simulink model "arquitetura"  (R2021a)
settings: Solver=VariableStepAuto  StartTime=0.0  StopTime=Ttotal  RelTol=1e-20
values from neighbouring files (symbols this model uses):
  r = R'*(current-reference)    [implemented_controller.m]
undefined symbols (not defined in the file or in its folder): def_seed, DiscIntNeverNeededParam, drone1_psi0, drone1_v0, drone1_x0, drone1_y0, drone2_psi0, drone2_v0, drone2_x0, drone2_y0, drone3_psi0, drone3_v0, drone3_x0, drone3_y0, gama_dot_constant, max_psi, max_vel, min_psi, min_vel, N, target_velocity, Ts, vel_target, vel_target_x, x0, y0
libraries: commrandsrc3 x2
settings Model: Creator=migue  LastModifiedBy=migue

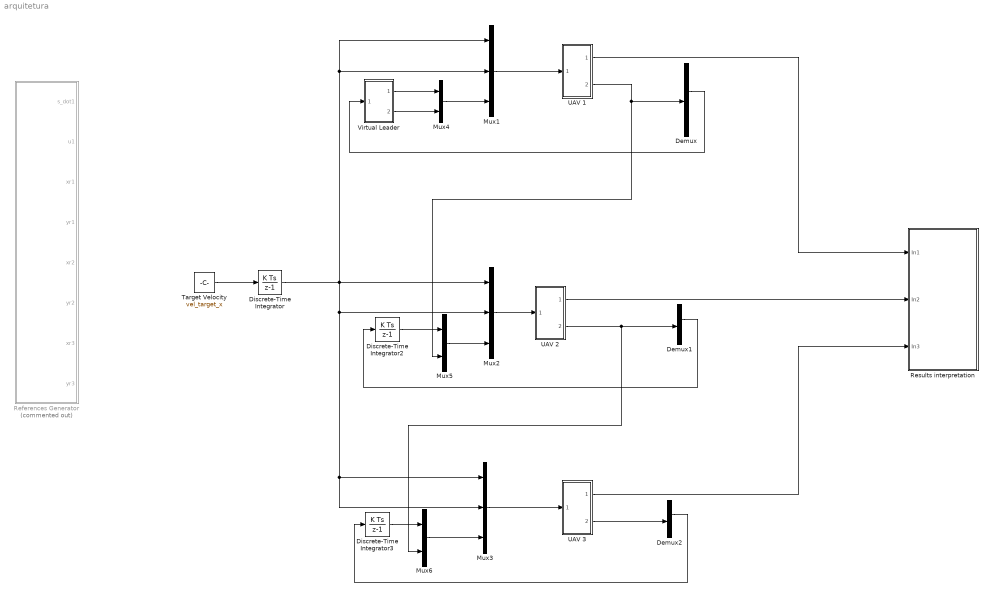
== system arquitetura ==
  Demux : Demux
  Demux1 : Demux
  Demux2 : Demux
  Discrete-Time Integrator : DiscreteIntegrator  SampleTime=Ts  ICPrevOutput=DiscIntNeverNeededParam  ICPrevScaledInput=DiscIntNeverNeededParam
  Discrete-Time Integrator2 : DiscreteIntegrator  SampleTime=Ts  ICPrevOutput=DiscIntNeverNeededParam  ICPrevScaledInput=DiscIntNeverNeededParam
  Discrete-Time Integrator3 : DiscreteIntegrator  SampleTime=Ts  ICPrevOutput=DiscIntNeverNeededParam  ICPrevScaledInput=DiscIntNeverNeededParam
  Mux1 : Mux  Inputs=3
  Mux2 : Mux  Inputs=3
  Mux3 : Mux  Inputs=3
  Mux4 : Mux  Inputs=2
  Mux5 : Mux  Inputs=2
  Mux6 : Mux  Inputs=2
  References Generator : Subsystem  Commented=on
  Results interpretation : Subsystem
  Target Velocity : Constant  Value=vel_target_x  SampleTime=Ts
  UAV 1 : Subsystem
  UAV 2 : Subsystem
  UAV 3 : Subsystem
  Virtual Leader : Subsystem
  wires:
  Mux1/1 -> UAV 1/1((x;y))
  Mux2/1 -> UAV 2/1((x;y))
  Mux3/1 -> UAV 3/1((x;y))
  Discrete-Time Integrator/1 -> Mux1/1, Mux1/2, Mux2/1, Mux3/2, Mux3/1, Mux2/2
  Target Velocity/1 -> Discrete-Time Integrator/1
  Mux4/1 -> Mux1/3
  UAV 1/2(Output) -> Demux/1, Mux5/2
  Discrete-Time Integrator2/1 -> Mux5/1
  Mux5/1 -> Mux2/3
  UAV 2/2(Output) -> Mux6/2, Demux1/1
  Mux6/1 -> Mux3/3
  Discrete-Time Integrator3/1 -> Mux6/1
  UAV 3/2(Output) -> Demux2/1
  UAV 1/1(Out1) -> Results interpretation/1(In1)
  UAV 2/1(Out1) -> Results interpretation/2(In2)
  UAV 3/1(Out1) -> Results interpretation/3(In3)
  Virtual Leader/1(Out1) -> Mux4/1
  Virtual Leader/2(Out2) -> Mux4/2
  Demux/2 -> Virtual Leader/1(Input)
  Demux1/2 -> Discrete-Time Integrator2/1
  Demux2/2 -> Discrete-Time Integrator3/1

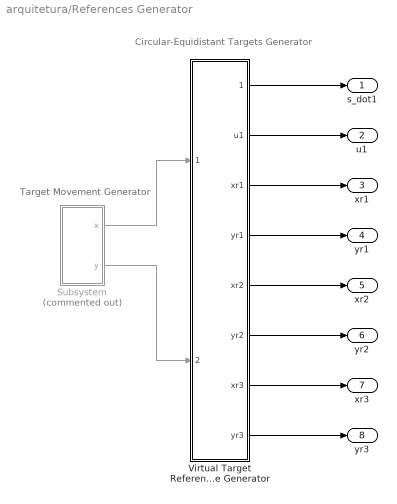
== system arquitetura/References Generator ==
  note: Target Movement Generator
  note: Circular-Equidistant Targets Generator
  Subsystem : Subsystem  Commented=on
  Virtual Target Reference Generator : Subsystem
  s_dot1 : Outport
  u1 : Outport  Port=2
  xr1 : Outport  Port=3
  yr1 : Outport  Port=4
  xr2 : Outport  Port=5
  yr2 : Outport  Port=6
  xr3 : Outport  Port=7
  yr3 : Outport  Port=8
  wires:
  Subsystem/2(y) -> Virtual Target Reference Generator/2(Input1)
  Subsystem/1(x) -> Virtual Target Reference Generator/1(Input)
  Virtual Target Reference Generator/4(yr1) -> yr1/1
  Virtual Target Reference Generator/6(yr2) -> yr2/1
  Virtual Target Reference Generator/3(xr1) -> xr1/1
  Virtual Target Reference Generator/5(xr2) -> xr2/1
  Virtual Target Reference Generator/8(yr3) -> yr3/1
  Virtual Target Reference Generator/7(xr3) -> xr3/1
  Virtual Target Reference Generator/2(u1) -> u1/1
  Virtual Target Reference Generator/1(s_dot1) -> s_dot1/1

== system arquitetura/Results interpretation ==
  In1 : Inport
  In2 : Inport  Port=2
  In3 : Inport  Port=3
  Draws Results : MATLABFcn  MATLABFcn=draw_results  OutputDimensions=0
  Mux : Mux  Inputs=3
  To Workspace : ToWorkspace  VariableName=simulation_data  SampleTime=-1
  wires:
  Mux/1 -> To Workspace/1, Draws Results/1
  In3/1 -> Mux/3
  In2/1 -> Mux/2
  In1/1 -> Mux/1

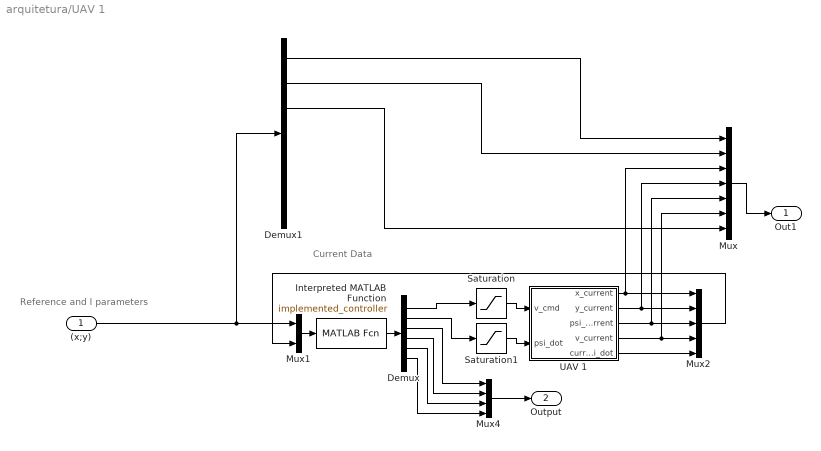
== system arquitetura/UAV 1 ==
  note: Current Data
  note: Reference and l parameters
  (x;y) : Inport
  Demux : Demux  Outputs=6
  Demux1 : Demux  Outputs=7
  Interpreted MATLAB Function : MATLABFcn  MATLABFcn=implemented_controller  OutputDimensions=6
  Mux : Mux  Inputs=7
  Mux1 : Mux  Inputs=2
  Mux2 : Mux  Inputs=5
  Mux4 : Mux
  Saturation : Saturate  UpperLimit=max_vel  LowerLimit=min_vel
  Saturation1 : Saturate  UpperLimit=max_psi  LowerLimit=min_psi
  UAV 1 : Subsystem
  Out1 : Outport
  Output : Outport  Port=2
  wires:
  Mux1/1 -> Interpreted MATLAB Function/1
  Interpreted MATLAB Function/1 -> Demux/1
  Demux/1 -> Saturation/1
  Saturation1/1 -> UAV 1/2(psi_dot)
  UAV 1/4(v_current) -> Mux/6, Mux2/4
  Mux2/1 -> Mux1/2
  Saturation/1 -> UAV 1/1(v_cmd)
  Demux/2 -> Saturation1/1
  (x;y)/1 -> Demux1/1, Mux1/1
  Demux1/1 -> Mux/1
  Demux1/2 -> Mux/2
  Mux/1 -> Out1/1
  UAV 1/3(psi_current) -> Mux/5, Mux2/3
  UAV 1/1(x_current) -> Mux/3, Mux2/1
  UAV 1/2(y_current) -> Mux/4, Mux2/2
  Demux/3 -> Mux4/1
  Demux/4 -> Mux4/2
  Mux4/1 -> Output/1
  Demux/5 -> Mux4/3
  Demux/6 -> Mux4/4
  UAV 1/5(current_psi_dot) -> Mux2/5
  Demux1/3 -> Mux/7

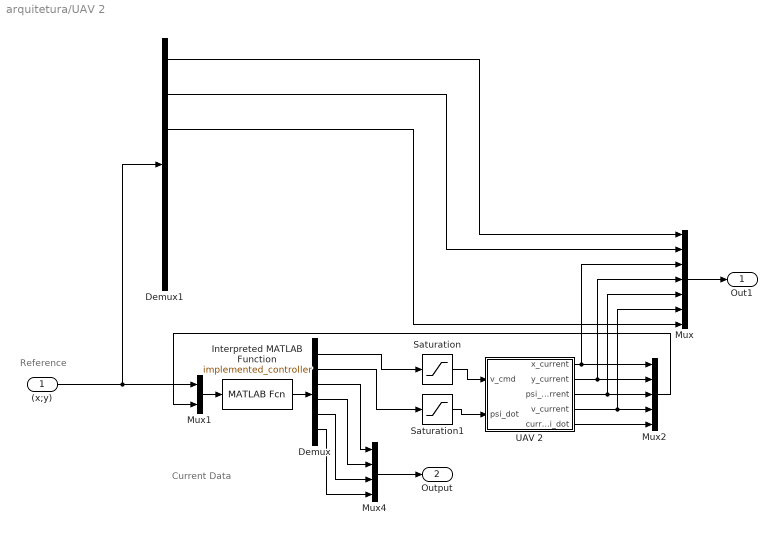
== system arquitetura/UAV 2 ==
  note: Current Data
  note: Reference
  (x;y) : Inport
  Demux : Demux  Outputs=6
  Demux1 : Demux  Outputs=7
  Interpreted MATLAB Function : MATLABFcn  MATLABFcn=implemented_controller  OutputDimensions=6
  Mux : Mux  Inputs=7
  Mux1 : Mux  Inputs=2
  Mux2 : Mux  Inputs=5
  Mux4 : Mux
  Saturation : Saturate  UpperLimit=max_vel  LowerLimit=min_vel
  Saturation1 : Saturate  UpperLimit=max_psi  LowerLimit=min_psi
  UAV 2 : Subsystem
  Out1 : Outport
  Output : Outport  Port=2
  wires:
  UAV 2/3(psi_current) -> Mux/5, Mux2/3
  Mux1/1 -> Interpreted MATLAB Function/1
  UAV 2/1(x_current) -> Mux2/1, Mux/3
  Interpreted MATLAB Function/1 -> Demux/1
  Demux/1 -> Saturation/1
  Saturation1/1 -> UAV 2/2(psi_dot)
  UAV 2/2(y_current) -> Mux/4, Mux2/2
  UAV 2/4(v_current) -> Mux/6, Mux2/4
  Mux2/1 -> Mux1/2
  Demux/2 -> Saturation1/1
  (x;y)/1 -> Demux1/1, Mux1/1
  Demux1/1 -> Mux/1
  Demux1/2 -> Mux/2
  Mux/1 -> Out1/1
  Mux4/1 -> Output/1
  Demux/3 -> Mux4/1
  Demux/4 -> Mux4/2
  Demux/5 -> Mux4/3
  Demux/6 -> Mux4/4
  Saturation/1 -> UAV 2/1(v_cmd)
  UAV 2/5(current_psi_dot) -> Mux2/5
  Demux1/3 -> Mux/7

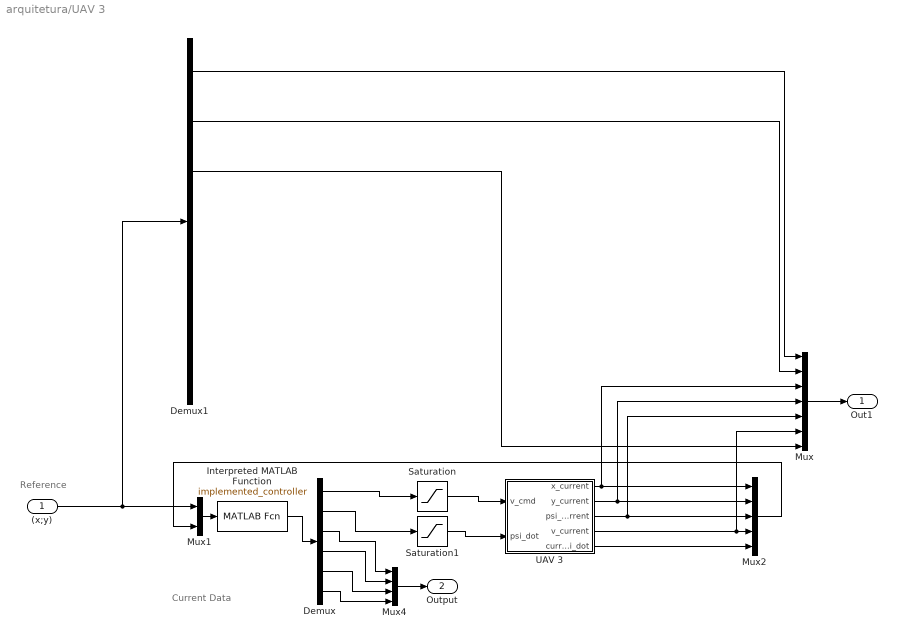
== system arquitetura/UAV 3 ==
  note: Current Data
  note: Reference
  (x;y) : Inport
  Demux : Demux  Outputs=6
  Demux1 : Demux  Outputs=7
  Interpreted MATLAB Function : MATLABFcn  MATLABFcn=implemented_controller  OutputDimensions=6
  Mux : Mux  Inputs=7
  Mux1 : Mux  Inputs=2
  Mux2 : Mux  Inputs=5
  Mux4 : Mux
  Saturation : Saturate  UpperLimit=max_vel  LowerLimit=min_vel
  Saturation1 : Saturate  UpperLimit=max_psi  LowerLimit=min_psi
  UAV 3 : Subsystem
  Out1 : Outport
  Output : Outport  Port=2
  wires:
  UAV 3/3(psi_current) -> Mux2/3, Mux/5
  Mux1/1 -> Interpreted MATLAB Function/1
  Interpreted MATLAB Function/1 -> Demux/1
  Demux/1 -> Saturation/1
  Saturation1/1 -> UAV 3/2(psi_dot)
  UAV 3/4(v_current) -> Mux2/4, Mux/6
  Mux2/1 -> Mux1/2
  Saturation/1 -> UAV 3/1(v_cmd)
  Demux/2 -> Saturation1/1
  (x;y)/1 -> Demux1/1, Mux1/1
  Demux1/1 -> Mux/1
  Demux1/2 -> Mux/2
  Mux/1 -> Out1/1
  UAV 3/1(x_current) -> Mux2/1, Mux/3
  UAV 3/2(y_current) -> Mux2/2, Mux/4
  Mux4/1 -> Output/1
  Demux/3 -> Mux4/1
  Demux/4 -> Mux4/2
  Demux/5 -> Mux4/3
  Demux/6 -> Mux4/4
  UAV 3/5(current_psi_dot) -> Mux2/5
  Demux1/3 -> Mux/7

== system arquitetura/Virtual Leader ==
  Input : Inport
  Constant2 : Constant  Value=0  SampleTime=Ts
  Constant4 : Constant  Value=15  SampleTime=Ts
  Discrete-Time Integrator1 : DiscreteIntegrator  SampleTime=Ts  ICPrevOutput=DiscIntNeverNeededParam  ICPrevScaledInput=DiscIntNeverNeededParam
  Discrete-Time Integrator2 : DiscreteIntegrator  SampleTime=Ts  ICPrevOutput=DiscIntNeverNeededParam  ICPrevScaledInput=DiscIntNeverNeededParam
  Mux7 : Mux
  Out1 : Outport
  Out2 : Outport  Port=2
  wires:
  Discrete-Time Integrator1/1 -> Out1/1
  Constant4/1 -> Discrete-Time Integrator2/1, Mux7/3, Mux7/2
  Constant2/1 -> Mux7/4
  Mux7/1 -> Out2/1
  Input/1 -> Discrete-Time Integrator1/1
  Discrete-Time Integrator2/1 -> Mux7/1

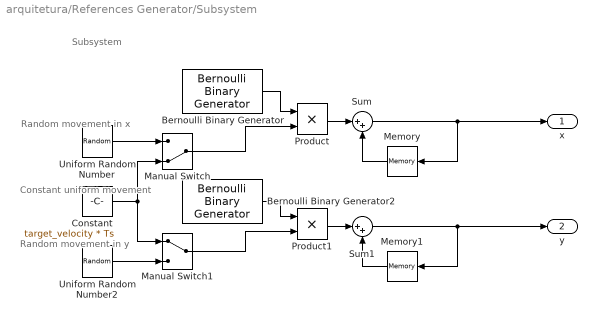
== system arquitetura/References Generator/Subsystem ==
  note: Random movement
      | in x
  note: Constant uniform
      | movement
  note: Subsystem
  note: Random movement
      | in y
  Bernoulli Binary Generator : commrandsrc3/Bernoulli Binary Generator  ProbabilityOfZero=probability_of_changing  SeedSource=Auto  Seed=0  SampleTime=Ts  SamplesPerFrame=1  OutputDataType=double  SimulateUsing=Interpreted execution
  Bernoulli Binary Generator2 : commrandsrc3/Bernoulli Binary Generator  ProbabilityOfZero=probability_of_changing  SeedSource=Auto  Seed=0  SampleTime=Ts  SamplesPerFrame=1  OutputDataType=double  SimulateUsing=Interpreted execution
  Constant : Constant  Value=target_velocity * Ts  SampleTime=Ts
  Manual Switch : ManualSwitch  CurrentSetting=0
  Manual Switch1 : ManualSwitch
  Memory : Memory  InitialCondition=x0
  Memory1 : Memory  InitialCondition=y0
  Product : Product
  Product1 : Product
  Sum : Sum  Inputs=|++
  Sum1 : Sum  Inputs=|++
  Uniform Random Number : UniformRandomNumber  Minimum=0  Maximum=3  Seed=def_seed  SampleTime=Ts
  Uniform Random Number2 : UniformRandomNumber  Minimum=0  Maximum=3  Seed=def_seed  SampleTime=Ts
  x : Outport
  y : Outport  Port=2
  wires:
  Constant/1 -> Manual Switch1/1, Manual Switch/2
  Uniform Random Number2/1 -> Manual Switch1/2
  Manual Switch1/1 -> Product1/2
  Manual Switch/1 -> Product/2
  Memory/1 -> Sum/2
  Memory1/1 -> Sum1/2
  Product1/1 -> Sum1/1
  Product/1 -> Sum/1
  Bernoulli Binary Generator2/1 -> Product1/1
  Sum/1 -> x/1, Memory/1
  Uniform Random Number/1 -> Manual Switch/1
  Sum1/1 -> Memory1/1, y/1
  Bernoulli Binary Generator/1 -> Product/1

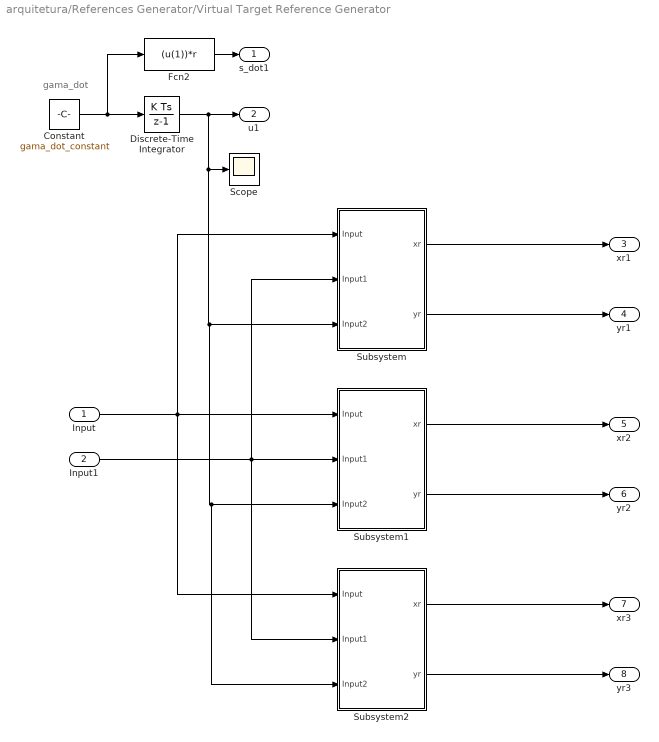
== system arquitetura/References Generator/Virtual Target Reference Generator ==
  note: gama_dot
  Input : Inport
  Input1 : Inport  Port=2
  Constant : Constant  Value=gama_dot_constant  SampleTime=Ts
  Discrete-Time Integrator : DiscreteIntegrator  SampleTime=Ts  ICPrevOutput=DiscIntNeverNeededParam  ICPrevScaledInput=DiscIntNeverNeededParam
  Fcn2 : Fcn  Expr=(u(1))*r
  Scope : Scope
  Subsystem : Subsystem
  Subsystem1 : Subsystem
  Subsystem2 : Subsystem
  s_dot1 : Outport  VectorParamsAs1DForOutWhenUnconnected=off
  u1 : Outport  Port=2  VectorParamsAs1DForOutWhenUnconnected=off
  xr1 : Outport  Port=3  VectorParamsAs1DForOutWhenUnconnected=off
  yr1 : Outport  Port=4  VectorParamsAs1DForOutWhenUnconnected=off
  xr2 : Outport  Port=5  VectorParamsAs1DForOutWhenUnconnected=off
  yr2 : Outport  Port=6  VectorParamsAs1DForOutWhenUnconnected=off
  xr3 : Outport  Port=7  VectorParamsAs1DForOutWhenUnconnected=off
  yr3 : Outport  Port=8  VectorParamsAs1DForOutWhenUnconnected=off
  wires:
  Subsystem/1(xr) -> xr1/1
  Subsystem/2(yr) -> yr1/1
  Subsystem1/1(xr) -> xr2/1
  Subsystem1/2(yr) -> yr2/1
  Input1/1 -> Subsystem2/2(Input1), Subsystem1/2(Input1), Subsystem/2(Input1)
  Input/1 -> Subsystem2/1(Input), Subsystem1/1(Input), Subsystem/1(Input)
  Subsystem2/1(xr) -> xr3/1
  Constant/1 -> Discrete-Time Integrator/1, Fcn2/1
  Discrete-Time Integrator/1 -> Scope/1, Subsystem2/3(Input2), Subsystem1/3(Input2), Subsystem/3(Input2), u1/1
  Fcn2/1 -> s_dot1/1
  Subsystem2/2(yr) -> yr3/1

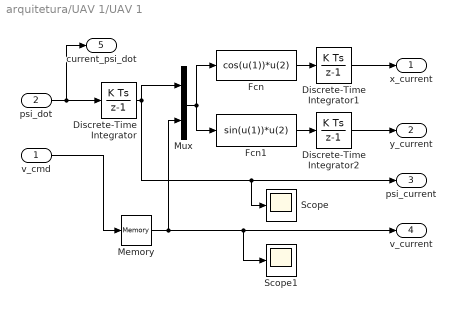
== system arquitetura/UAV 1/UAV 1 ==
  v_cmd : Inport
  psi_dot : Inport  Port=2
  Discrete-Time Integrator : DiscreteIntegrator  InitialCondition=drone1_psi0  SampleTime=Ts  ICPrevOutput=DiscIntNeverNeededParam  ICPrevScaledInput=DiscIntNeverNeededParam
  Discrete-Time Integrator1 : DiscreteIntegrator  InitialCondition=drone1_x0  SampleTime=Ts  ICPrevOutput=DiscIntNeverNeededParam  ICPrevScaledInput=DiscIntNeverNeededParam
  Discrete-Time Integrator2 : DiscreteIntegrator  InitialCondition=drone1_y0  SampleTime=Ts  ICPrevOutput=DiscIntNeverNeededParam  ICPrevScaledInput=DiscIntNeverNeededParam
  Fcn : Fcn  Expr=cos(u(1))*u(2)
  Fcn1 : Fcn  Expr=sin(u(1))*u(2)
  Memory : Memory  InitialCondition=drone1_v0
  Mux : Mux  Inputs=2
  Scope : Scope
  Scope1 : Scope
  x_current : Outport  VectorParamsAs1DForOutWhenUnconnected=off
  y_current : Outport  Port=2  VectorParamsAs1DForOutWhenUnconnected=off
  psi_current : Outport  Port=3  VectorParamsAs1DForOutWhenUnconnected=off
  v_current : Outport  Port=4  VectorParamsAs1DForOutWhenUnconnected=off
  current_psi_dot : Outport  Port=5
  wires:
  Discrete-Time Integrator1/1 -> x_current/1
  Discrete-Time Integrator2/1 -> y_current/1
  Fcn/1 -> Discrete-Time Integrator1/1
  Fcn1/1 -> Discrete-Time Integrator2/1
  psi_dot/1 -> current_psi_dot/1, Discrete-Time Integrator/1
  Mux/1 -> Fcn/1, Fcn1/1
  v_cmd/1 -> Memory/1
  Discrete-Time Integrator/1 -> Mux/1, Scope/1, psi_current/1
  Memory/1 -> Scope1/1, v_current/1, Mux/2

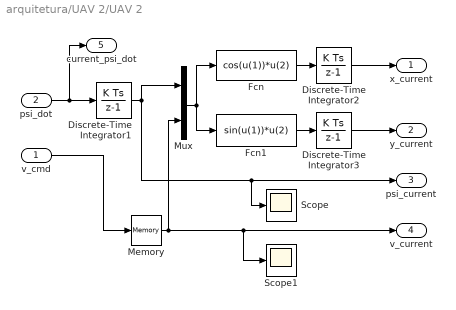
== system arquitetura/UAV 2/UAV 2 ==
  v_cmd : Inport
  psi_dot : Inport  Port=2
  Discrete-Time Integrator1 : DiscreteIntegrator  InitialCondition=drone2_psi0  SampleTime=Ts  ICPrevOutput=DiscIntNeverNeededParam  ICPrevScaledInput=DiscIntNeverNeededParam
  Discrete-Time Integrator2 : DiscreteIntegrator  InitialCondition=drone2_x0  SampleTime=Ts  ICPrevOutput=DiscIntNeverNeededParam  ICPrevScaledInput=DiscIntNeverNeededParam
  Discrete-Time Integrator3 : DiscreteIntegrator  InitialCondition=drone2_y0  SampleTime=Ts  ICPrevOutput=DiscIntNeverNeededParam  ICPrevScaledInput=DiscIntNeverNeededParam
  Fcn : Fcn  Expr=cos(u(1))*u(2)
  Fcn1 : Fcn  Expr=sin(u(1))*u(2)
  Memory : Memory  InitialCondition=drone2_v0
  Mux : Mux  Inputs=2
  Scope : Scope
  Scope1 : Scope
  x_current : Outport  VectorParamsAs1DForOutWhenUnconnected=off
  y_current : Outport  Port=2  VectorParamsAs1DForOutWhenUnconnected=off
  psi_current : Outport  Port=3  VectorParamsAs1DForOutWhenUnconnected=off
  v_current : Outport  Port=4  VectorParamsAs1DForOutWhenUnconnected=off
  current_psi_dot : Outport  Port=5
  wires:
  Discrete-Time Integrator2/1 -> x_current/1
  Discrete-Time Integrator3/1 -> y_current/1
  Fcn/1 -> Discrete-Time Integrator2/1
  Fcn1/1 -> Discrete-Time Integrator3/1
  psi_dot/1 -> current_psi_dot/1, Discrete-Time Integrator1/1
  Mux/1 -> Fcn/1, Fcn1/1
  v_cmd/1 -> Memory/1
  Discrete-Time Integrator1/1 -> Mux/1, Scope/1, psi_current/1
  Memory/1 -> Scope1/1, v_current/1, Mux/2

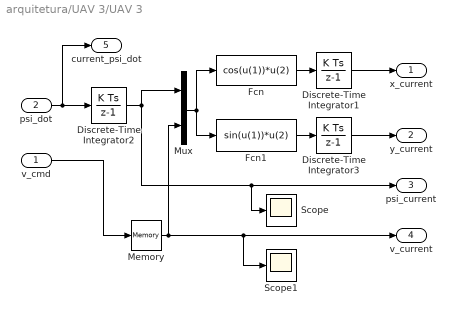
== system arquitetura/UAV 3/UAV 3 ==
  v_cmd : Inport
  psi_dot : Inport  Port=2
  Discrete-Time Integrator1 : DiscreteIntegrator  InitialCondition=drone3_x0  SampleTime=Ts  ICPrevOutput=DiscIntNeverNeededParam  ICPrevScaledInput=DiscIntNeverNeededParam
  Discrete-Time Integrator2 : DiscreteIntegrator  InitialCondition=drone3_psi0  SampleTime=Ts  ICPrevOutput=DiscIntNeverNeededParam  ICPrevScaledInput=DiscIntNeverNeededParam
  Discrete-Time Integrator3 : DiscreteIntegrator  InitialCondition=drone3_y0  SampleTime=Ts  ICPrevOutput=DiscIntNeverNeededParam  ICPrevScaledInput=DiscIntNeverNeededParam
  Fcn : Fcn  Expr=cos(u(1))*u(2)
  Fcn1 : Fcn  Expr=sin(u(1))*u(2)
  Memory : Memory  InitialCondition=drone3_v0
  Mux : Mux  Inputs=2
  Scope : Scope
  Scope1 : Scope
  x_current : Outport  VectorParamsAs1DForOutWhenUnconnected=off
  y_current : Outport  Port=2  VectorParamsAs1DForOutWhenUnconnected=off
  psi_current : Outport  Port=3  VectorParamsAs1DForOutWhenUnconnected=off
  v_current : Outport  Port=4  VectorParamsAs1DForOutWhenUnconnected=off
  current_psi_dot : Outport  Port=5
  wires:
  Discrete-Time Integrator1/1 -> x_current/1
  Discrete-Time Integrator3/1 -> y_current/1
  Fcn/1 -> Discrete-Time Integrator1/1
  Fcn1/1 -> Discrete-Time Integrator3/1
  psi_dot/1 -> current_psi_dot/1, Discrete-Time Integrator2/1
  Mux/1 -> Fcn/1, Fcn1/1
  v_cmd/1 -> Memory/1
  Discrete-Time Integrator2/1 -> Mux/1, Scope/1, psi_current/1
  Memory/1 -> Scope1/1, v_current/1, Mux/2

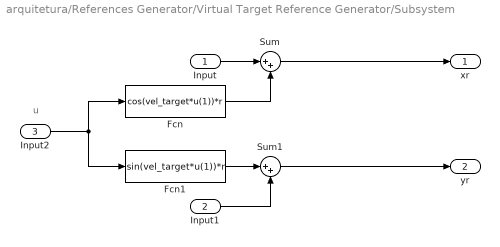
== system arquitetura/References Generator/Virtual Target Reference Generator/Subsystem ==
  note: u
  Input : Inport
  Input1 : Inport  Port=2
  Input2 : Inport  Port=3
  Fcn : Fcn  Expr=cos(vel_target*u(1))*r
  Fcn1 : Fcn  Expr=sin(vel_target*u(1))*r
  Sum : Sum  Inputs=|++
  Sum1 : Sum  Inputs=|++
  xr : Outport  VectorParamsAs1DForOutWhenUnconnected=off
  yr : Outport  Port=2  VectorParamsAs1DForOutWhenUnconnected=off
  wires:
  Fcn/1 -> Sum/2
  Input/1 -> Sum/1
  Sum1/1 -> yr/1
  Sum/1 -> xr/1
  Input1/1 -> Sum1/2
  Fcn1/1 -> Sum1/1
  Input2/1 -> Fcn1/1, Fcn/1

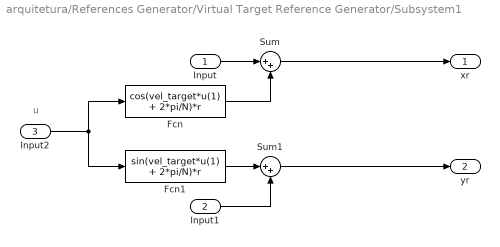
== system arquitetura/References Generator/Virtual Target Reference Generator/Subsystem1 ==
  note: u
  Input : Inport
  Input1 : Inport  Port=2
  Input2 : Inport  Port=3
  Fcn : Fcn  Expr=cos(vel_target*u(1) + 2*pi/N)*r
  Fcn1 : Fcn  Expr=sin(vel_target*u(1) + 2*pi/N)*r
  Sum : Sum  Inputs=|++
  Sum1 : Sum  Inputs=|++
  xr : Outport  VectorParamsAs1DForOutWhenUnconnected=off
  yr : Outport  Port=2  VectorParamsAs1DForOutWhenUnconnected=off
  wires:
  Fcn/1 -> Sum/2
  Input/1 -> Sum/1
  Sum1/1 -> yr/1
  Sum/1 -> xr/1
  Input1/1 -> Sum1/2
  Fcn1/1 -> Sum1/1
  Input2/1 -> Fcn1/1, Fcn/1

== system arquitetura/References Generator/Virtual Target Reference Generator/Subsystem2 ==
  note: u
  Input : Inport
  Input1 : Inport  Port=2
  Input2 : Inport  Port=3
  Fcn : Fcn  Expr=cos(vel_target*u(1) + (2*2*pi)/N)*r
  Fcn1 : Fcn  Expr=sin(vel_target*u(1) + (2*2*pi)/N)*r
  Sum : Sum  Inputs=|++
  Sum1 : Sum  Inputs=|++
  xr : Outport  VectorParamsAs1DForOutWhenUnconnected=off
  yr : Outport  Port=2  VectorParamsAs1DForOutWhenUnconnected=off
  wires:
  Fcn/1 -> Sum/2
  Input/1 -> Sum/1
  Sum1/1 -> yr/1
  Sum/1 -> xr/1
  Input1/1 -> Sum1/2
  Fcn1/1 -> Sum1/1
  Input2/1 -> Fcn1/1, Fcn/1
